simulink model "lin_propulsion"  (R2016b)
settings: Solver=VariableStepAuto  StartTime=0.0  StopTime=250  RelTol=1e-3
values from neighbouring files (symbols this model uses):
  a = -5.4036    [lin_propulsion_params.m]    (also in robust_lin_propulsion_params_zs.m; ship_induction_motor_propulsion_extended_linear.m)
  b = -3.499    [lin_propulsion_params.m]    (also in robust_lin_propulsion_params_zs.m; ship_induction_motor_propulsion_extended_linear.m)
  g = -0.5816    [lin_propulsion_params.m]    (also in robust_lin_propulsion_params_zs.m; ship_induction_motor_propulsion_extended_linear.m)
  Ki = 1    [lin_propulsion_params.m]    (also in robust_lin_propulsion_params_zs.m; ship_induction_motor_propulsion_extended_linear.m)
  Kp = 2    [lin_propulsion_params.m]    (also in robust_lin_propulsion_params_zs.m; ship_induction_motor_propulsion_extended_linear.m)
  p = 6.58    [lin_propulsion_params.m]    (also in robust_lin_propulsion_params_zs.m; ship_induction_motor_propulsion_extended_linear.m)
  q = 5.0245    [lin_propulsion_params.m]    (also in robust_lin_propulsion_params_zs.m; ship_induction_motor_propulsion_extended_linear.m)
  Tn = 7.83    [lin_propulsion_params.m]    (also in robust_lin_propulsion_params_zs.m; ship_induction_motor_propulsion_extended_linear.m)
  Tth = 2    [lin_propulsion_params.m]    (also in robust_lin_propulsion_params_zs.m; ship_induction_motor_propulsion_extended_linear.m)
  Tv = 115.69    [lin_propulsion_params.m]    (also in robust_lin_propulsion_params_zs.m; ship_induction_motor_propulsion_extended_linear.m)
  v = 1.9099    [lin_propulsion_params.m]    (also in robust_lin_propulsion_params_zs.m; ship_induction_motor_propulsion_extended_linear.m)
libraries: simulink x1
settings Model: Creator=z003vh9b  LastModifiedBy=z003vh9b

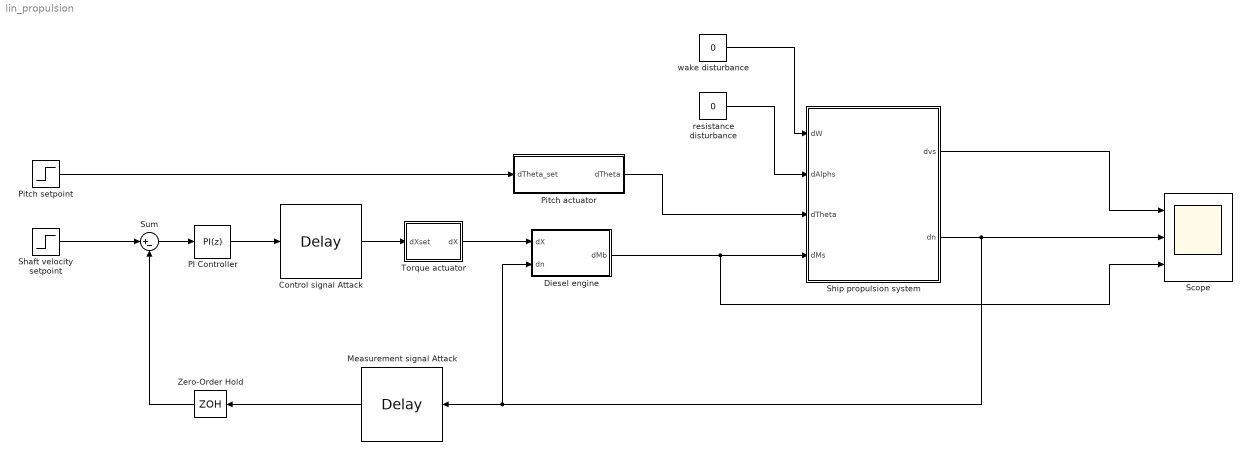
== system lin_propulsion ==
  Control signal Attack : TransportDelay  DelayTime=0
  Diesel engine : Subsystem
  Measurement signal Attack : TransportDelay  DelayTime=[0 5]
  PI Controller : simulink/Continuous/PID Controller  Controller=PI  TimeDomain=Discrete-time  SampleTime=1  IntegratorMethod=Forward Euler  FilterMethod=Forward Euler  Form=Parallel  UseFilter=on  ControllerParametersSource=internal  P=Kp  I=Ki  D=0  N=100  InitialConditionSource=internal  InitialConditionForIntegrator=0  InitialConditionForFilter=0  ExternalReset=none  LimitOutput=off  UpperSaturationLimit=inf  LowerSaturationLimit=-inf  LinearizeAsGain=on  AntiWindupMode=none  Kb=1  TrackingMode=off  Kt=1  PParamMin=[]  PParamMax=[]  IParamMin=[]  IParamMax=[]  DParamMin=[]  DParamMax=[]  NParamMin=[]  NParamMax=[]  KbParamMin=[]  KbParamMax=[]  KtParamMin=[]  KtParamMax=[]  POutMin=[]  POutMax=[]  IOutMin=[]  IOutMax=[]  DOutMin=[]  DOutMax=[]  NOutMin=[]  NOutMax=[]  KbOutMin=[]  KbOutMax=[]  KtOutMin=[]  KtOutMax=[]  IntegratorOutMin=[]  IntegratorOutMax=[]  FilterOutMin=[]  FilterOutMax=[]  SumOutMin=[]  SumOutMax=[]  SumI1OutMin=[]  SumI1OutMax=[]  SumI2OutMin=[]  SumI2OutMax=[]  SumI3OutMin=[]  SumI3OutMax=[]  SumDOutMin=[]  SumDOutMax=[]  SaturationOutMin=[]  SaturationOutMax=[]  IntegratorContinuousStateAttributes=''  IntegratorStateMustResolveToSignalObject=off  IntegratorRTWStateStorageClass=Auto  FilterContinuousStateAttributes=''  FilterStateMustResolveToSignalObject=off  FilterRTWStateStorageClass=Auto  DifferentiatorICPrevScaledInput=0  DifferentiatorOutMin=[]  DifferentiatorOutMax=[]
  Pitch actuator : Subsystem
  Pitch setpoint : Step  Time=150  After=-0.05  SampleTime=0
  Scope : Scope  NumInputPorts=3
  Shaft velocity setpoint : Step  Time=100  After=0.1  SampleTime=0
  Ship propulsion system : Subsystem
  Sum : Sum  Inputs=|+-
  Torque actuator : Subsystem
  Zero-Order Hold : ZeroOrderHold
  resistance disturbance : Constant  Value=0
  wake disturbance : Constant  Value=0
  wires:
  Diesel engine/1(dMb) -> Scope/3, Ship propulsion system/4(dMs)
  Torque actuator/1(dX) -> Diesel engine/1(dX)
  Sum/1 -> PI Controller/1
  Pitch actuator/1(dTheta) -> Ship propulsion system/3(dTheta)
  Pitch setpoint/1 -> Pitch actuator/1(dTheta_set)
  Shaft velocity setpoint/1 -> Sum/1
  Ship propulsion system/1(dvs) -> Scope/1
  resistance disturbance/1 -> Ship propulsion system/2(dAlphs)
  wake disturbance/1 -> Ship propulsion system/1(dW)
  PI Controller/1 -> Control signal Attack/1
  Ship propulsion system/2(dn) -> Diesel engine/2(dn), Measurement signal Attack/1, Scope/2
  Control signal Attack/1 -> Torque actuator/1(dXset)
  Zero-Order Hold/1 -> Sum/2
  Measurement signal Attack/1 -> Zero-Order Hold/1

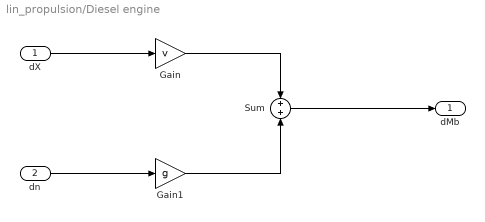
== system lin_propulsion/Diesel engine ==
  dX : Inport
  dn : Inport  Port=2
  Gain : Gain  Gain=v
  Gain1 : Gain  Gain=g
  Sum : Sum
  dMb : Outport
  wires:
  dX/1 -> Gain/1
  dn/1 -> Gain1/1
  Gain/1 -> Sum/1
  Gain1/1 -> Sum/2
  Sum/1 -> dMb/1

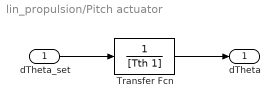
== system lin_propulsion/Pitch actuator ==
  dTheta_set : Inport
  Transfer Fcn : TransferFcn  Denominator=[Tth 1]
  dTheta : Outport
  wires:
  dTheta_set/1 -> Transfer Fcn/1
  Transfer Fcn/1 -> dTheta/1

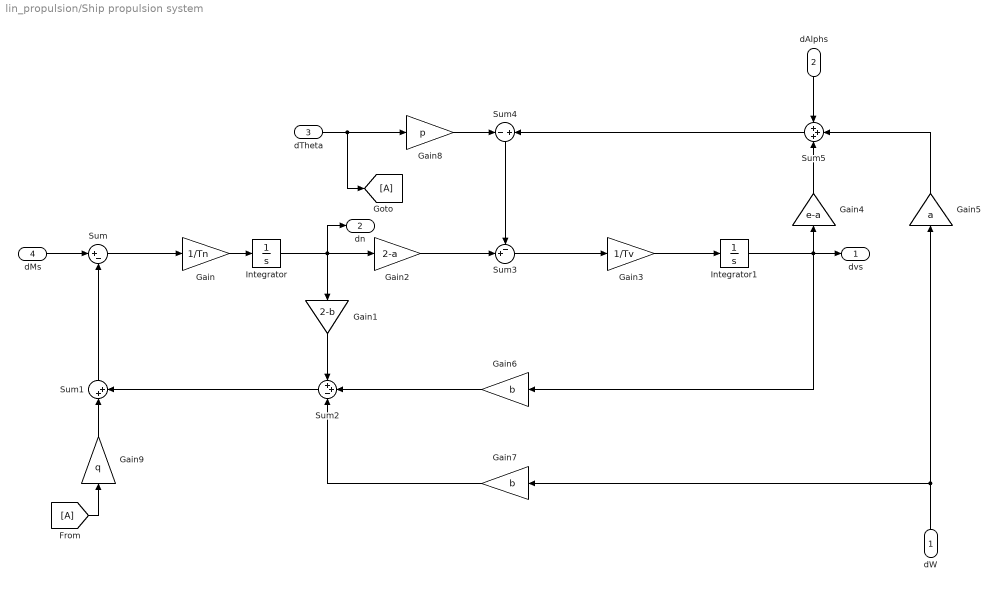
== system lin_propulsion/Ship propulsion system ==
  dW : Inport
  dAlphs : Inport  Port=2
  dTheta : Inport  Port=3
  dMs : Inport  Port=4
  Gain : Gain  Gain=1/Tn
  Gain1 : Gain  Gain=2-b
  Gain2 : Gain  Gain=2-a
  Gain3 : Gain  Gain=1/Tv
  Gain4 : Gain  Gain=e-a
  Gain5 : Gain  Gain=a
  Gain6 : Gain  Gain=b
  Gain7 : Gain  Gain=b
  Gain8 : Gain  Gain=p
  Gain9 : Gain  Gain=q
  Integrator : Integrator
  Integrator1 : Integrator
  Sum : Sum  Inputs=|+-
  Sum1 : Sum  Inputs=|++
  Sum2 : Sum  Inputs=++-
  Sum3 : Sum  Inputs=-+|
  Sum4 : Sum  Inputs=-+
  Sum5 : Sum  Inputs=+++
  dvs : Outport
  dn : Outport  Port=2
  wires:
  Sum1/1 -> Sum/2
  Sum/1 -> Gain/1
  Gain/1 -> Integrator/1
  Integrator/1 -> dn/1, Gain1/1, Gain2/1
  Gain2/1 -> Sum3/2
  Sum4/1 -> Sum3/1
  Sum3/1 -> Gain3/1
  Gain8/1 -> Sum4/1
  Sum5/1 -> Sum4/2
  Gain4/1 -> Sum5/3
  Integrator1/1 -> dvs/1, Gain6/1, Gain4/1
  Gain3/1 -> Integrator1/1
  Gain5/1 -> Sum5/2
  Gain7/1 -> Sum2/3
  Gain6/1 -> Sum2/2
  Gain1/1 -> Sum2/1
  Sum2/1 -> Sum1/2
  Gain9/1 -> Sum1/1
  dW/1 -> Gain5/1, Gain7/1
  dAlphs/1 -> Sum5/1
  dTheta/1 -> [A], Gain8/1
  [A] -> Gain9/1
  dMs/1 -> Sum/1

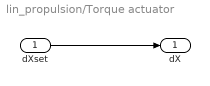
== system lin_propulsion/Torque actuator ==
  dXset : Inport
  dX : Outport
  wires:
  dXset/1 -> dX/1
